simulink model "Assgn_1_18EE35014_Part_1"  (R2020b)
settings: Solver=VariableStepAuto  StartTime=0.0  StopTime=0.004  RelTol=1e-9
settings Model: Creator=Pratyush Jaiswal  LastModifiedBy=Pratyush Jaiswal

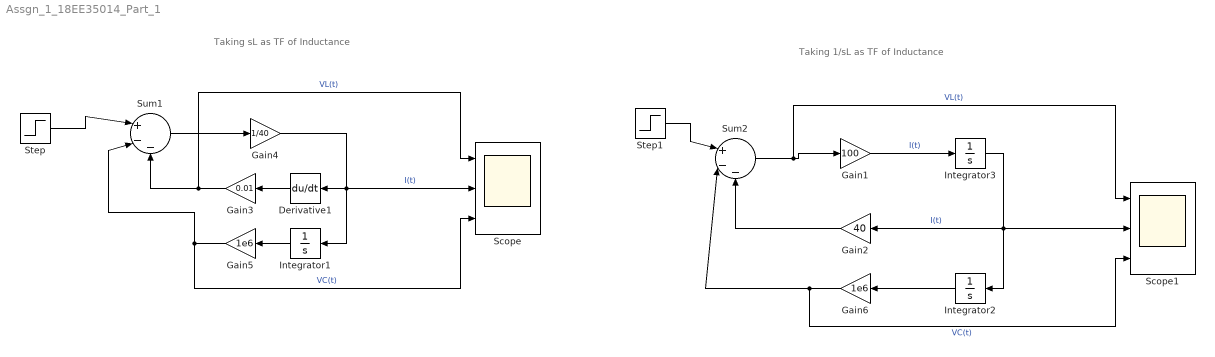
== system Assgn_1_18EE35014_Part_1 ==
  note: Taking sL as TF of Inductance
  note: Taking 1/sL as TF of Inductance
  Derivative1 : Derivative
  Gain1 : Gain  Gain=100
  Gain2 : Gain  Gain=40
  Gain3 : Gain  Gain=0.01
  Gain4 : Gain  Gain=1/40
  Gain5 : Gain  Gain=1e6
  Gain6 : Gain  Gain=1e6
  Integrator1 : Integrator
  Integrator2 : Integrator
  Integrator3 : Integrator
  Scope : Scope  NumInputPorts=3
  Scope1 : Scope  NumInputPorts=3
  Step : Step  Time=0  SampleTime=0  ZeroCross=off
  Step1 : Step  Time=0  SampleTime=0  ZeroCross=off
  Sum1 : Sum  Inputs=|+--
  Sum2 : Sum  Inputs=|+--
  wires:
  Gain5/1 -> Scope/3, Sum1/2  "VC(t)"
  Integrator1/1 -> Gain5/1
  Gain4/1 -> Scope/2, Derivative1/1, Integrator1/1  "I(t)"
  Sum1/1 -> Gain4/1
  Derivative1/1 -> Gain3/1
  Gain3/1 -> Scope/1, Sum1/3  "VL(t)"
  Step/1 -> Sum1/1
  Step1/1 -> Sum2/1
  Gain2/1 -> Sum2/3
  Gain6/1 -> Scope1/3, Sum2/2  "VC(t)"
  Integrator2/1 -> Gain6/1
  Gain1/1 -> Integrator3/1  "I(t)"
  Sum2/1 -> Scope1/1, Gain1/1  "VL(t)"
  Integrator3/1 -> Scope1/2, Integrator2/1, Gain2/1  "I(t)"
